simulink model "obse"  (R2020a)
settings: Solver=VariableStepAuto  StartTime=0.0  StopTime=5.0  RelTol=1e-3
values from neighbouring files (symbols this model uses):
  K1 = real(K1)    [observa.m]
  L2 = real(L2)    [observa.m]
undefined symbols (not defined in the file or in its folder): A, B, C, x0
settings Model: Creator=wyton  LastModifiedBy=wyton

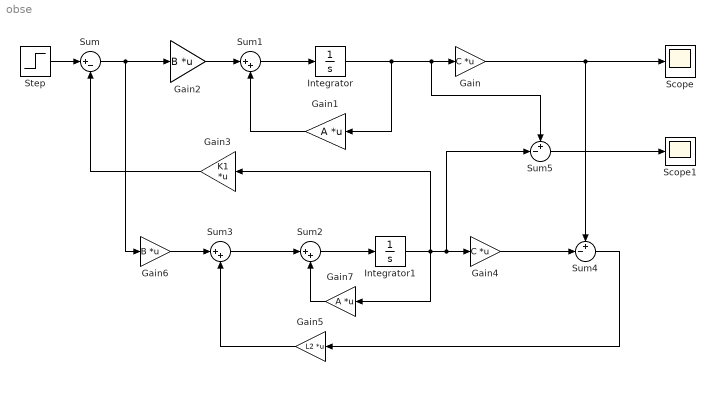
== system obse ==
  Gain : Gain  Gain=C  Multiplication=Matrix(K*u)
      settings: AttributesFormatString=C
  Gain1 : Gain  Gain=A  Multiplication=Matrix(K*u)
      settings: AttributesFormatString=A
  Gain2 : Gain  Tag=B  Gain=B  Multiplication=Matrix(K*u)
      settings: AttributesFormatString=B
  Gain3 : Gain  Gain=K1  Multiplication=Matrix(K*u)
      settings: AttributesFormatString=K
  Gain4 : Gain  Gain=C  Multiplication=Matrix(K*u)
      settings: AttributesFormatString=C
  Gain5 : Gain  Gain=L2  Multiplication=Matrix(K*u)
      settings: AttributesFormatString=L
  Gain6 : Gain  Gain=B  Multiplication=Matrix(K*u)
      settings: AttributesFormatString=B
  Gain7 : Gain  Gain=A  Multiplication=Matrix(K*u)
      settings: AttributesFormatString=A
  Integrator : Integrator  InitialCondition=x0
  Integrator1 : Integrator
  Scope : Scope
      settings: AttributesFormatString=output
  Scope1 : Scope
      settings: AttributesFormatString=state error
  Step : Step  Time=0  Before=[0,0]  After=[0;0]  SampleTime=0
  Sum : Sum  Inputs=|+-
  Sum1 : Sum  Inputs=|++
  Sum2 : Sum  Inputs=|++
  Sum3 : Sum  Inputs=|++
  Sum4 : Sum  Inputs=+-|
  Sum5 : Sum  Inputs=+-|
  wires:
  Step/1 -> Sum/1
  Sum/1 -> Gain6/1, Gain2/1
  Sum1/1 -> Integrator/1
  Gain2/1 -> Sum1/1
  Integrator/1 -> Gain1/1, Sum5/1, Gain/1
  Gain1/1 -> Sum1/2
  Gain/1 -> Sum4/1, Scope/1
  Gain3/1 -> Sum/2
  Gain6/1 -> Sum3/1
  Gain5/1 -> Sum3/2
  Sum3/1 -> Sum2/1
  Gain7/1 -> Sum2/2
  Sum2/1 -> Integrator1/1
  Integrator1/1 -> Gain3/1, Sum5/2, Gain4/1, Gain7/1
  Gain4/1 -> Sum4/2
  Sum5/1 -> Scope1/1
  Sum4/1 -> Gain5/1
